simulink model "with_Parasitics"  (R2024a)
settings: Solver=VariableStepAuto  StartTime=0.0  StopTime=1  RelTol=1e-3
libraries: spsSeriesRLCBranchLib x12, spsCurrentMeasurementLib x1, spsDiodeLib x1, spsDCVoltageSourceLib x1, spsMosfetLib x1, spsVoltageMeasurementLib x1, sps_lib x1
settings Model: Creator=AEES-STUDENT  LastModifiedBy=AEES-STUDENT
settings SolverCC: ZeroCrossAlgorithm=Adaptive
settings DebuggingCC: IgnoredZcDiagnostic=none

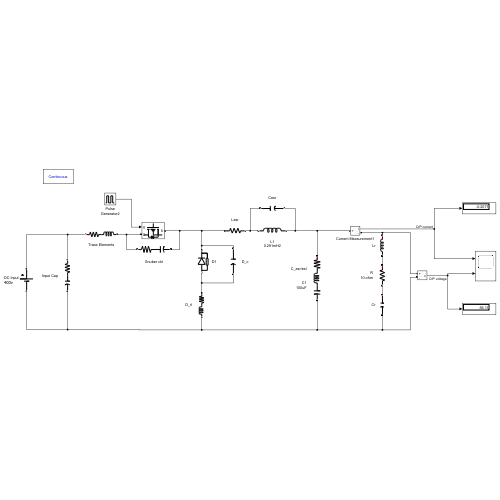
[thumbnail: Simulink's stored preview of the top-level diagram]
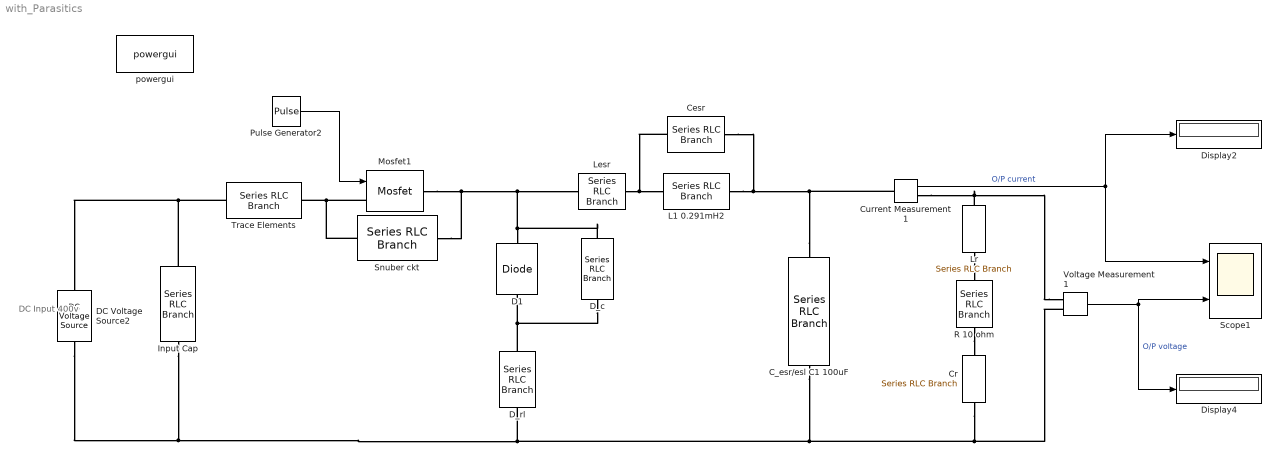
== system with_Parasitics ==
  note: DC Input
      | 400v
  C_esr/esl C1 100uF : spsSeriesRLCBranchLib/Series RLC Branch  LConnTagsString=__new0  RConnTagsString=__new0  BranchType=RLC  Resistance=10e-3  Inductance=10e-9  SetiL0=off  InitialCurrent=0  Capacitance=100e-6  Setx0=off  InitialVoltage=0  Measurements=None
  Cesr : spsSeriesRLCBranchLib/Series RLC Branch  LConnTagsString=__new0  RConnTagsString=__new0  BranchType=C  Resistance=0.1  Inductance=0.291e-3  SetiL0=off  InitialCurrent=0  Capacitance=10e-12  Setx0=off  InitialVoltage=0  Measurements=None
  Cr : spsSeriesRLCBranchLib/Series RLC Branch  LConnTagsString=__new0  RConnTagsString=__new0  BranchType=C  Resistance=10  Inductance=10e-9  SetiL0=off  InitialCurrent=0  Capacitance=10e-12  Setx0=off  InitialVoltage=0  Measurements=None
  Current Measurement1 : spsCurrentMeasurementLib/Current Measurement  PhasorSimulation=off  OutputType=Complex  PSBequivalent=0
  D1 : spsDiodeLib/Diode  Ron=0.001  Lon=0  Vf=0.8  IC=0  UseSnubber=0  Rs=500  Cs=250e-9  Measurements=off
  DC Voltage Source2 : spsDCVoltageSourceLib/DC Voltage Source  Amplitude=400  Measurements=None
  D_c : spsSeriesRLCBranchLib/Series RLC Branch  LConnTagsString=__new0  RConnTagsString=__new0  BranchType=C  Resistance=0.1  Inductance=0.291e-3  SetiL0=off  InitialCurrent=0  Capacitance=5e-12  Setx0=off  InitialVoltage=0  Measurements=None
  D_rl : spsSeriesRLCBranchLib/Series RLC Branch  LConnTagsString=__new0  RConnTagsString=__new0  BranchType=RL  Resistance=0.5  Inductance=10e-9  SetiL0=off  InitialCurrent=0  Capacitance=100e-6  Setx0=off  InitialVoltage=0  Measurements=None
  Display2 : Display
  Display4 : Display
  Input Cap : spsSeriesRLCBranchLib/Series RLC Branch  LConnTagsString=__new0  RConnTagsString=__new0  BranchType=RC  Resistance=10e-3  Inductance=0.1e-12  SetiL0=off  InitialCurrent=0  Capacitance=1e-6  Setx0=off  InitialVoltage=0  Measurements=None
  L1 0.291mH2 : spsSeriesRLCBranchLib/Series RLC Branch  LConnTagsString=__new0  RConnTagsString=__new0  BranchType=L  Resistance=100e-3  Inductance=0.291e-3  SetiL0=off  InitialCurrent=0  Capacitance=1e-6  Setx0=off  InitialVoltage=0  Measurements=None
  Lesr : spsSeriesRLCBranchLib/Series RLC Branch  LConnTagsString=__new0  RConnTagsString=__new0  BranchType=R  Resistance=10e-3  Inductance=1e-3  SetiL0=off  InitialCurrent=0  Capacitance=100e-6  Setx0=off  InitialVoltage=0  Measurements=None
  Lr : spsSeriesRLCBranchLib/Series RLC Branch  LConnTagsString=__new0  RConnTagsString=__new0  BranchType=L  Resistance=10  Inductance=10e-9  SetiL0=off  InitialCurrent=0  Capacitance=100e-6  Setx0=off  InitialVoltage=0  Measurements=None
  Mosfet1 : spsMosfetLib/Mosfet  Ron=0.03  Lon=0  Rd=0.03  Vfd=1.2  IC=0  Rs=9  Cs=1e-9  Measurements=off
  Pulse Generator2 : DiscretePulseGenerator  PulseType=Time based  Amplitude=15  Period=1/200000  PulseWidth=3.147
  R 10 ohm : spsSeriesRLCBranchLib/Series RLC Branch  LConnTagsString=__new0  RConnTagsString=__new0  BranchType=R  Resistance=10  Inductance=1e-3  SetiL0=off  InitialCurrent=0  Capacitance=100e-6  Setx0=off  InitialVoltage=0  Measurements=None
  Scope1 : Scope  NumInputPorts=2
  Snuber ckt : spsSeriesRLCBranchLib/Series RLC Branch  LConnTagsString=__new0  RConnTagsString=__new0  BranchType=RC  Resistance=0.01  Inductance=0.291e-3  SetiL0=off  InitialCurrent=0  Capacitance=50e-12  Setx0=off  InitialVoltage=0  Measurements=None
  Trace Elements : spsSeriesRLCBranchLib/Series RLC Branch  LConnTagsString=__new0  RConnTagsString=__new0  BranchType=RL  Resistance=0.1e-9  Inductance=10e-9  SetiL0=off  InitialCurrent=0  Capacitance=100e-6  Setx0=off  InitialVoltage=0  Measurements=None
  Voltage Measurement1 : spsVoltageMeasurementLib/Voltage Measurement  PhasorSimulation=off  OutputType=Complex  PSBequivalent=0
  powergui : sps_lib/powergui  Priority=1  SimulationMode=Continuous  SampleTime=50e-6  frequency=60  Iterations=50  frequencyindice=0  Pbase=100e6  ErrMax=1e-4  UnitsV=kV  UnitsW=MW  buscounter=0  FunctionMessages=off  echomessages=off  EnableUseOfTLC=off  CurrentSourceSwitches=off  DisableSnubberDevices=off  DisableRonSwitches=off  DisableVfSwitches=off  DisplayEquations=off  AutomaticDiscreteSolvers=off  SolverType=Tustin/Backward Euler (TBE)  Interpol=off  ExternalGateDelay=off  methode=off  Ts=100  x0status=blocks  SPID=on  SwTol=0  HookPort=off  NonlinearTolerance=1e-4  nMaxIteration=100  ContinueOnMaxIteration=off  RestoreLinks=warning  ResistiveCurrentMeasurement=off  Frange=[0:2:500]  Ylog=off  Xlog=on  ShowGrid=off  save=off  variable=ZData  structure=0  ZoomFFT=off  StartTime=0.0  cycles=1  DisplayStyle=1  fundamental=60  FreqAxis=off  MaxFrequency=1000  frequencyindicesteady=1  RmsSteady=1  display=off
  wires:
  Pulse Generator2/1 -> Mosfet1/1
  Voltage Measurement1/1 -> Scope1/2, Display4/1  "O/P voltage"
  Current Measurement1/1 -> Display2/1, Scope1/1  "O/P current"
  connections:
  Voltage Measurement1/LConn2 -- Cr/RConn1 -- C_esr/esl C1 100uF/RConn1 -- Input Cap/RConn1 -- DC Voltage Source2/LConn1 -- D_rl/RConn1
  C_esr/esl C1 100uF/LConn1 -- Current Measurement1/LConn1 -- Cesr/RConn1 -- L1 0.291mH2/RConn1
  D1/RConn1 -- Snuber ckt/RConn1 -- Mosfet1/RConn1 -- Lesr/LConn1 -- D_c/LConn1
  Voltage Measurement1/LConn1 -- Lr/LConn1 -- Current Measurement1/RConn1
  Mosfet1/LConn1 -- Snuber ckt/LConn1 -- Trace Elements/RConn1
  D_rl/LConn1 -- D_c/RConn1 -- D1/LConn1
  Trace Elements/LConn1 -- DC Voltage Source2/RConn1 -- Input Cap/LConn1
  Lr/RConn1 -- R 10 ohm/LConn1
  R 10 ohm/RConn1 -- Cr/LConn1
  Lesr/RConn1 -- Cesr/LConn1 -- L1 0.291mH2/LConn1
